simulink model "clik_inverse"  (Simulink 10.2)
settings: Solver=ode1  StartTime=0.0  StopTime=4  FixedStep=0.001  RelTol=1e-3
undefined symbols (not defined in the file or in its folder): DiscIntNeverNeededParam, q0, Tc
settings Model: Creator=Xp  LastModifiedBy=Megha
settings DataIOCC: LimitDataPoints=on
settings OptimizationCC: ExpressionDepthLimit=2147483647  InitFltsAndDblsToZero=on
settings DebuggingCC: SaveWithParameterizedLinksMsg=none  SolverPrmCheckMsg=warning  MultiTaskDSMMsg=warning  MultiTaskCondExecSysMsg=none  StateNameClashWarn=warning
settings SFSimCC: SimUseLocalCustomCode=on
settings RTWCC: RTWUseLocalCustomCode=on
settings ConfigComp: CovExternalEMLEnable=on

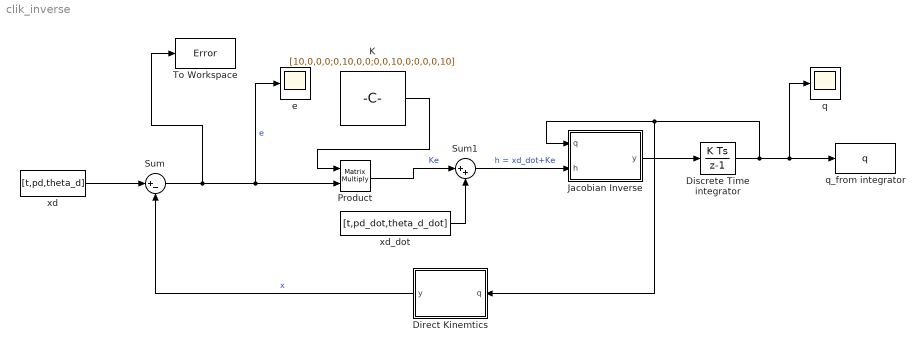
== system clik_inverse ==
  Direct Kinemtics : MATLAB Function  TreatAsAtomicUnit=on
  Discrete Time integrator : DiscreteIntegrator  InitialCondition=q0  SampleTime=Tc  ICPrevOutput=DiscIntNeverNeededParam  ICPrevScaledInput=DiscIntNeverNeededParam
  Jacobian Inverse : MATLAB Function  TreatAsAtomicUnit=on
  K : Constant  Value=[10,0,0,0;0,10,0,0;0,0,10,0;0,0,0,10]
  Product : Product  Multiplication=Matrix(*)
  Sum : Sum  Inputs=|+-
  Sum1 : Sum  Inputs=|++
  To Workspace : ToWorkspace  VariableName=Error  SaveFormat=Timeseries  SampleTime=-1
  e : Scope
  q : Scope
  q_from integrator : ToWorkspace  VariableName=q  SaveFormat=Timeseries  SampleTime=-1
  xd : FromWorkspace  VariableName=[t,pd,theta_d]
  xd_dot : FromWorkspace  VariableName=[t,pd_dot,theta_d_dot]
  wires:
  Jacobian Inverse/1(y) -> Discrete Time integrator/1
  K/1 -> Product/1
  Product/1 -> Sum1/1  "Ke"
  xd/1 -> Sum/1
  xd_dot/1 -> Sum1/2
  Sum1/1 -> Jacobian Inverse/2(h)  "h = xd_dot+Ke"
  Direct Kinemtics/1(y) -> Sum/2  "x"
  Discrete Time integrator/1 -> q_from integrator/1, q/1, Jacobian Inverse/1(q), Direct Kinemtics/1(q)
  Sum/1 -> To Workspace/1, e/1, Product/2  "e"

== matlab function Jacobian Inverse ==
  data: q input double; y output double; h input double
function y = fcn(q,h)

theta_1 = q(1);
theta_2 = q(2);
d3 = q(3);
theta_4  = q(4);
j11 = (2*(cos(theta_1)*cos(theta_2) - sin(theta_1)*sin(theta_2)))/(sin(theta_2)*cos(theta_1)^2 + sin(theta_2)*sin(theta_1)^2);
j12 = (2*(cos(theta_1)*sin(theta_2) + cos(theta_2)*sin(theta_1)))/(sin(theta_2)*cos(theta_1)^2 + sin(theta_2)*sin(theta_1)^2);
j13 = 0; 
j14 = 0;

j21 = -(2*(cos(theta_1) + cos(theta_1)*cos(theta_2) - sin(theta_1)*sin(theta_2)))/(sin(theta_2)*cos(theta_1)^2 + sin(theta_2)*sin(theta_1)^2);
j22 = -(2*(sin(theta_1) + cos(theta_1)*sin(theta_2) + cos(theta_2)*sin(theta_1)))/(sin(theta_2)*cos(theta_1)^2 + sin(theta_2)*sin(theta_1)^2);
j23 = 0;
j24 = 0;

j31 = 0;
j32 = 0;
j33 = -1;
j34 = 0;

j41 = (2*cos(theta_1))/(sin(theta_2)*cos(theta_1)^2 + sin(theta_2)*sin(theta_1)^2);
j42 = (2*sin(theta_1))/(sin(theta_2)*cos(theta_1)^2 + sin(theta_2)*sin(theta_1)^2);
j43 = 0;
j44 = 1;

J_inv = [j11,j12,j13,j14;j21,j22,j23,j24;j31,j32,j33,j34;j41,j42,j43,j44];
q_dot = J_inv * h;
y = q_dot;

== matlab function Direct Kinemtics ==
  data: q input double; y output double
function y = fcn(q)
q
theta_1 = q(1);
theta_2 = q(2);
d3 = q(3);
theta_4 = q(4);
t14 = cos(theta_1)/2 + (cos(theta_1)*cos(theta_2))/2 - (sin(theta_1)*sin(theta_2))/2;
t24 = sin(theta_1)/2 + (cos(theta_1)*sin(theta_2))/2 + (cos(theta_2)*sin(theta_1))/2;
t34 = 1-d3;
pe = [t14;t24;t34];
phi = (theta_1 + theta_2 + theta_4);
xe =[pe;phi];
y = xe;
